simulink model "VehicleModel"  (R2020b)
settings: Solver=FixedStepAuto  StartTime=0.0  StopTime=1068  FixedStep=0.1  RelTol=1e-3
model workspace (MAT data in the model file):
  t : mpt.Parameter (value not decoded)
(part 5 of 5)

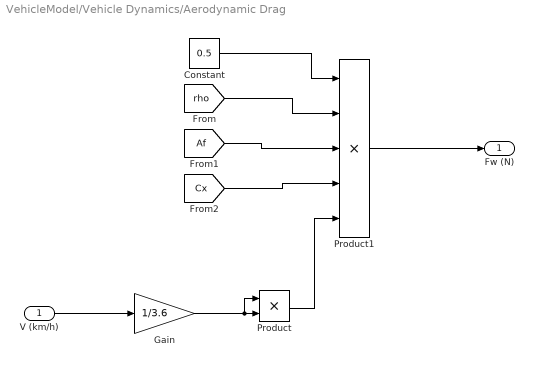
== system VehicleModel/Vehicle Dynamics/Aerodynamic Drag ==
  V (km/h) : Inport
  Constant : Constant  Value=0.5
  Gain : Gain  Gain=1/3.6
  Product : Product
  Product1 : Product  Inputs=5
  Fw (N) : Outport
  wires:
  Product1/1 -> Fw (N)/1
  Constant/1 -> Product1/1
  Gain/1 -> Product/1, Product/2
  Product/1 -> Product1/5
  V (km/h)/1 -> Gain/1
  [rho] -> Product1/2
  [Af] -> Product1/3
  [Cx] -> Product1/4

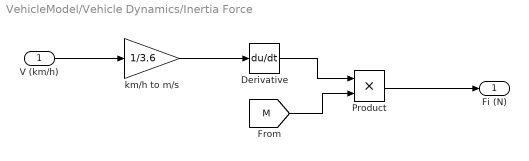
== system VehicleModel/Vehicle Dynamics/Inertia Force ==
  V (km/h) : Inport
  Derivative : Derivative
  Product : Product
  km/h to m/s : Gain  Gain=1/3.6
  Fi (N) : Outport
  wires:
  km/h to m/s/1 -> Derivative/1
  Product/1 -> Fi (N)/1
  V (km/h)/1 -> km/h to m/s/1
  Derivative/1 -> Product/1
  [M] -> Product/2

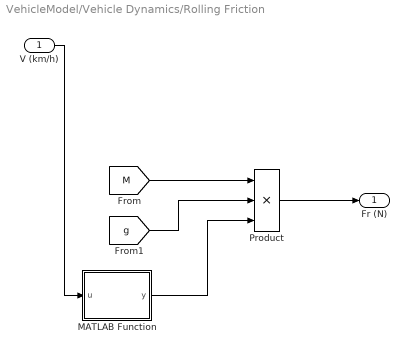
== system VehicleModel/Vehicle Dynamics/Rolling Friction ==
  V (km/h) : Inport
  MATLAB Function : MATLAB Function  TreatAsAtomicUnit=on
  Product : Product  Inputs=3
  Fr (N) : Outport
  wires:
  V (km/h)/1 -> MATLAB Function/1(u)
  MATLAB Function/1(y) -> Product/3
  Product/1 -> Fr (N)/1
  [M] -> Product/1
  [g] -> Product/2

== matlab function VehicleModel/Vehicle Dynamics/Rolling Friction/MATLAB Function ==
  data: u input; y output
function y = fcn(u)

y = 0.01*(1+u/100);
